simulink subsystem "runsum"  (R2020b)
settings: Solver=VariableStepAuto  StartTime=0.0  StopTime=10.0  RelTol=1e-3
settings Model: DefaultTestHarness=runsum_Harness1  Creator=IIT_KGP_CSE_FM_LAB  LastModifiedBy=IIT_KGP_CSE_FM_LAB

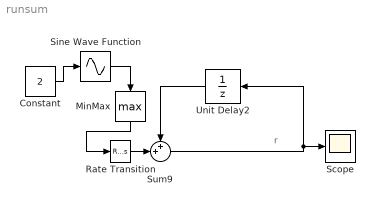
== system runsum ==
  note: r
  Constant : Constant  Value=2
  MinMax : MinMax  Function=max
  Rate Transition : RateTransition
  Scope : Scope
  Sine Wave Function : Sin  TimeSource=Use external signal  SampleTime=0
  Sum9 : Sum  Inputs=++|
  Unit Delay2 : UnitDelay  SampleTime=-1  HasFrameUpgradeWarning=on
  wires:
  Unit Delay2/1 -> Sum9/1
  Sum9/1 -> Scope/1, Unit Delay2/1
  Rate Transition/1 -> Sum9/2
  Constant/1 -> Sine Wave Function/1
  Sine Wave Function/1 -> MinMax/1
  MinMax/1 -> Rate Transition/1
